simulink model "trial"  (R2015b)
settings: Solver=VariableStepAuto  StartTime=0.0  StopTime=10.0  RelTol=1e-3
undefined symbols (not defined in the file or in its folder): Ts, Ts_IO601
libraries: dspswit3 x1, simulink_extras x1
settings Model: Creator=1SMARTe  LastModifiedBy=1SMARTe

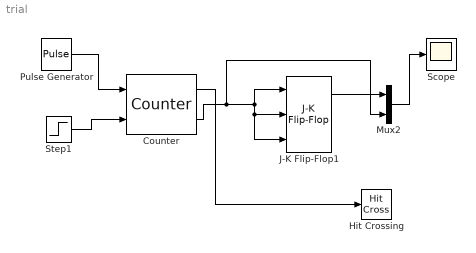
== system trial ==
  Counter : dspswit3/Counter  Direction=Up  CountEvent=Rising edge  CounterSize=User defined  MaxCount=15  InitialCount=0  Output=Count and Hit  HitValue=5  ResetInput=on  SamplesPerFrame=1  Ts=1  CntDtype=double  HitDtype=Boolean
  Hit Crossing : HitCross  HitCrossingOffset=5  HitCrossingDirection=rising  ZeroCross=off
  J-K Flip-Flop1 : simulink_extras/Flip Flops/J-K Flip-Flop  initial_condition=0
  Mux2 : Mux  Inputs=2
  Pulse Generator : DiscretePulseGenerator  PulseType=Time based  Period=Ts*10  PulseWidth=10  SampleTime=Ts_IO601
  Scope : Scope
  Step1 : Step  Time=3  SampleTime=Ts
  wires:
  Step1/1 -> Counter/2
  Pulse Generator/1 -> Counter/1
  Counter/2 -> Mux2/2, J-K Flip-Flop1/2, J-K Flip-Flop1/3, J-K Flip-Flop1/1
  Counter/1 -> Hit Crossing/1
  J-K Flip-Flop1/1 -> Mux2/1
  Mux2/1 -> Scope/1
